simulink library "ammclib_bam_S32K14x"  (R2016a)
settings: Solver=VariableStepAuto  SolverMode=SingleTasking  StartTime=0.0  StopTime=10.0  RelTol=1e-3
undefined symbols (not defined in the file or in its folder): f16A1, f16A2, f16ADCMaxError, f16B0, f16B1, f16B2, f16C1, f16CC1, f16CC1sc, f16CC1sc_D, f16CC1sc_Q, f16CC2, f16CC2sc, f16CC2sc_D, f16CC2sc_Q, f16DerivGain, f16EGain, f16FiltCoef, f16HystOff, f16HystOn, f16IGain, f16IntegGain, f16IntegGainFW, f16IntegGainQ, f16Kd, f16Kq, f16Limit, f16LowerLimit, f16LowerLimit_D, f16LowerLimit_Q, f16LowerLimitFW, f16LowerLimitQ, f16ModIndex, f16OutValOff, f16OutValOn, f16PropGain, f16PropGainFW, f16PropGainQ, f16RampDown, f16RampUp, f16UGain, f16UpperLimit, f16UpperLimit_D, f16UpperLimit_Q, f16UpperLimitFW, f16UpperLimitQ, f16WIGain, f32A1, f32A2, f32ADCMaxError, f32B0, f32B1, f32B2, f32C1, f32CC1, f32CC1sc, f32CC1sc_D, f32CC1sc_Q, f32CC2, f32CC2sc ... (+114)
(part 20 of 22)

== system ammclib_bam_S32K14x/GMCLIB/F16/GMCLIB_DecouplingPMSM_F16 ==
  pUdq : Inport  OutDataTypeStr=Bus: SWLIBS_2Syst_F16  BusOutputAsStruct=on
  pIdq : Inport  Port=2  OutDataTypeStr=Bus: SWLIBS_2Syst_F16  BusOutputAsStruct=on
  f16AngularVel : Inport  Port=3  OutDataTypeStr=int16
  GMCLIB_DecouplingPMSM_SF : S-Function  FunctionName=GMCLIB_DecouplingPMSM_SF_F16  Parameters=showStates,f16Kd,s16KdShift,f16Kq,s16KqShift  SFunctionDeploymentMode=off  EnableBusSupport=off
  copyright : Subsystem
      mask Display: text(10,90,'FILE:');text(10,75,'DESRIPTION:');text(10,60,'COPYRIGHT:');text(10,45,'VERSION:');text(10,30,'DATE:')
  copyright2 : Subsystem
      mask Display: text(10,90,'GMCLIB_DecouplingPMSM_BAM_F16.mdl');text(10,75,'Decoupling of d and q axis of PMSM model.');text(10,60,'NXP 2020');text(10,45,'1.0');text(10,30,'24-Mar-2020');
  f16Kd : Ground
  f16Kq : Ground
  s16KdShift : Ground
  s16KqShift : Ground
  pUdqDec : Outport
  wires:
  GMCLIB_DecouplingPMSM_SF/1 -> pUdqDec/1
  s16KqShift/1 -> GMCLIB_DecouplingPMSM_SF/7
  f16Kq/1 -> GMCLIB_DecouplingPMSM_SF/6
  s16KdShift/1 -> GMCLIB_DecouplingPMSM_SF/5
  f16Kd/1 -> GMCLIB_DecouplingPMSM_SF/4
  f16AngularVel/1 -> GMCLIB_DecouplingPMSM_SF/3
  pIdq/1 -> GMCLIB_DecouplingPMSM_SF/2
  pUdq/1 -> GMCLIB_DecouplingPMSM_SF/1

== system ammclib_bam_S32K14x/GMCLIB/F16/GMCLIB_ElimDcBusRip_F16 ==
  pIn : Inport  OutDataTypeStr=Bus: SWLIBS_2Syst_F16  BusOutputAsStruct=on
  f16ArgDcBusMsr : Inport  Port=2  OutDataTypeStr=int16
  GMCLIB_ElimDcBusRip_SF : S-Function  FunctionName=GMCLIB_ElimDcBusRip_SF_F16  Parameters=showStates,f16ModIndex  SFunctionDeploymentMode=off  EnableBusSupport=off
  copyright : Subsystem
      mask Display: text(10,90,'FILE:');text(10,75,'DESRIPTION:');text(10,60,'COPYRIGHT:');text(10,45,'VERSION:');text(10,30,'DATE:')
  copyright2 : Subsystem
      mask Display: text(10,90,'GMCLIB_ElimDcBusRip_BAM_F16.mdl');text(10,75,'DC Bus voltage ripple elimination function.');text(10,60,'NXP 2020');text(10,45,'1.0');text(10,30,'18-Mar-2020');
  f16ModIndex : Ground
  pOut : Outport
  wires:
  GMCLIB_ElimDcBusRip_SF/1 -> pOut/1
  f16ModIndex/1 -> GMCLIB_ElimDcBusRip_SF/3
  f16ArgDcBusMsr/1 -> GMCLIB_ElimDcBusRip_SF/2
  pIn/1 -> GMCLIB_ElimDcBusRip_SF/1

== system ammclib_bam_S32K14x/GMCLIB/F16/GMCLIB_ParkInv_F16 ==
  pInAngle : Inport  OutDataTypeStr=Bus: SWLIBS_2Syst_F16  BusOutputAsStruct=on
  pIn : Inport  Port=2  OutDataTypeStr=Bus: SWLIBS_2Syst_F16  BusOutputAsStruct=on
  GMCLIB_ParkInv_SF : S-Function  FunctionName=GMCLIB_ParkInv_SF_F16  SFunctionDeploymentMode=off  EnableBusSupport=off
  copyright : Subsystem
      mask Display: text(10,90,'FILE:');text(10,75,'DESRIPTION:');text(10,60,'COPYRIGHT:');text(10,45,'VERSION:');text(10,30,'DATE:')
  copyright2 : Subsystem
      mask Display: text(10,90,'GMCLIB_ParkInv_BAM_F16.mdl');text(10,75,'Inverse Park transformation.');text(10,60,'NXP 2020');text(10,45,'1.0');text(10,30,'18-Mar-2020');
  pOut : Outport
  wires:
  GMCLIB_ParkInv_SF/1 -> pOut/1
  pIn/1 -> GMCLIB_ParkInv_SF/2
  pInAngle/1 -> GMCLIB_ParkInv_SF/1

== system ammclib_bam_S32K14x/GMCLIB/F16/GMCLIB_Park_F16 ==
  pInAngle : Inport  OutDataTypeStr=Bus: SWLIBS_2Syst_F16  BusOutputAsStruct=on
  pIn : Inport  Port=2  OutDataTypeStr=Bus: SWLIBS_2Syst_F16  BusOutputAsStruct=on
  GMCLIB_Park_SF : S-Function  FunctionName=GMCLIB_Park_SF_F16  SFunctionDeploymentMode=off  EnableBusSupport=off
  copyright : Subsystem
      mask Display: text(10,90,'FILE:');text(10,75,'DESRIPTION:');text(10,60,'COPYRIGHT:');text(10,45,'VERSION:');text(10,30,'DATE:')
  copyright2 : Subsystem
      mask Display: text(10,90,'GMCLIB_Park_BAM_F16.mdl');text(10,75,'Park transformation.');text(10,60,'NXP 2020');text(10,45,'1.0');text(10,30,'18-Mar-2020');
  pOut : Outport
  wires:
  GMCLIB_Park_SF/1 -> pOut/1
  pIn/1 -> GMCLIB_Park_SF/2
  pInAngle/1 -> GMCLIB_Park_SF/1

== system ammclib_bam_S32K14x/GMCLIB/F16/GMCLIB_PwmIct_F16 ==
  pIn : Inport  OutDataTypeStr=Bus: SWLIBS_2Syst_F16  BusOutputAsStruct=on
  GMCLIB_PwmIct_SF : S-Function  FunctionName=GMCLIB_PwmIct_SF_F16  SFunctionDeploymentMode=off  EnableBusSupport=off
  copyright : Subsystem
      mask Display: text(10,90,'FILE:');text(10,75,'DESRIPTION:');text(10,60,'COPYRIGHT:');text(10,45,'VERSION:');text(10,30,'DATE:')
  copyright2 : Subsystem
      mask Display: text(10,90,'GMCLIB_PwmIct_BAM_F16.mdl');text(10,75,'General Sinusoidal PWM.');text(10,60,'NXP 2020');text(10,45,'1.0');text(10,30,'18-Mar-2020');
  u16Sector : Outport
  pOut : Outport  Port=2
  wires:
  GMCLIB_PwmIct_SF/2 -> pOut/1
  GMCLIB_PwmIct_SF/1 -> u16Sector/1
  pIn/1 -> GMCLIB_PwmIct_SF/1

== system ammclib_bam_S32K14x/GMCLIB/F16/GMCLIB_SvmSci_F16 ==
  pIn : Inport  OutDataTypeStr=Bus: SWLIBS_2Syst_F16  BusOutputAsStruct=on
  GMCLIB_SvmSci_SF : S-Function  FunctionName=GMCLIB_SvmSci_SF_F16  SFunctionDeploymentMode=off  EnableBusSupport=off
  copyright : Subsystem
      mask Display: text(10,90,'FILE:');text(10,75,'DESRIPTION:');text(10,60,'COPYRIGHT:');text(10,45,'VERSION:');text(10,30,'DATE:')
  copyright2 : Subsystem
      mask Display: text(10,90,'GMCLIB_SvmSci_BAM_F16.mdl');text(10,75,'General Sinusoidal Modulation with Injection of Third Harmonic.');text(10,60,'NXP 2020');text(10,45,'1.0');text(10,30,'18-Mar-2020');
  u16Sector : Outport
  pOut : Outport  Port=2
  wires:
  GMCLIB_SvmSci_SF/2 -> pOut/1
  GMCLIB_SvmSci_SF/1 -> u16Sector/1
  pIn/1 -> GMCLIB_SvmSci_SF/1

== system ammclib_bam_S32K14x/GMCLIB/F16/GMCLIB_SvmStd_F16 ==
  pIn : Inport  OutDataTypeStr=Bus: SWLIBS_2Syst_F16  BusOutputAsStruct=on
  GMCLIB_SvmStd_SF : S-Function  FunctionName=GMCLIB_SvmStd_SF_F16  SFunctionDeploymentMode=off  EnableBusSupport=off
  copyright : Subsystem
      mask Display: text(10,90,'FILE:');text(10,75,'DESRIPTION:');text(10,60,'COPYRIGHT:');text(10,45,'VERSION:');text(10,30,'DATE:')
  copyright2 : Subsystem
      mask Display: text(10,90,'GMCLIB_SvmStd_BAM_F16.mdl');text(10,75,'Standard Space Vector Modulation.');text(10,60,'NXP 2020');text(10,45,'1.0');text(10,30,'18-Mar-2020');
  u16Sector : Outport
  pOut : Outport  Port=2
  wires:
  GMCLIB_SvmStd_SF/2 -> pOut/1
  GMCLIB_SvmStd_SF/1 -> u16Sector/1
  pIn/1 -> GMCLIB_SvmStd_SF/1

== system ammclib_bam_S32K14x/GMCLIB/F16/GMCLIB_SvmU0n_F16 ==
  pIn : Inport  OutDataTypeStr=Bus: SWLIBS_2Syst_F16  BusOutputAsStruct=on
  GMCLIB_SvmU0n_SF : S-Function  FunctionName=GMCLIB_SvmU0n_SF_F16  SFunctionDeploymentMode=off  EnableBusSupport=off
  copyright : Subsystem
      mask Display: text(10,90,'FILE:');text(10,75,'DESRIPTION:');text(10,60,'COPYRIGHT:');text(10,45,'VERSION:');text(10,30,'DATE:')
  copyright2 : Subsystem
      mask Display: text(10,90,'GMCLIB_SvmU0n_BAM_F16.mdl');text(10,75,'Special Space Vector Modulation with O_000 Nulls.');text(10,60,'NXP 2020');text(10,45,'1.0');text(10,30,'18-Mar-2020');
  u16Sector : Outport
  pOut : Outport  Port=2
  wires:
  GMCLIB_SvmU0n_SF/2 -> pOut/1
  GMCLIB_SvmU0n_SF/1 -> u16Sector/1
  pIn/1 -> GMCLIB_SvmU0n_SF/1

== system ammclib_bam_S32K14x/GMCLIB/F16/GMCLIB_SvmU7n_F16 ==
  pIn : Inport  OutDataTypeStr=Bus: SWLIBS_2Syst_F16  BusOutputAsStruct=on
  GMCLIB_SvmU7n_SF : S-Function  FunctionName=GMCLIB_SvmU7n_SF_F16  SFunctionDeploymentMode=off  EnableBusSupport=off
  copyright : Subsystem
      mask Display: text(10,90,'FILE:');text(10,75,'DESRIPTION:');text(10,60,'COPYRIGHT:');text(10,45,'VERSION:');text(10,30,'DATE:')
  copyright2 : Subsystem
      mask Display: text(10,90,'GMCLIB_SvmU7n_BAM_F16.mdl');text(10,75,'Special Space Vector Modulation with O_111 Ones.');text(10,60,'NXP 2020');text(10,45,'1.0');text(10,30,'18-Mar-2020');
  u16Sector : Outport
  pOut : Outport  Port=2
  wires:
  GMCLIB_SvmU7n_SF/2 -> pOut/1
  GMCLIB_SvmU7n_SF/1 -> u16Sector/1
  pIn/1 -> GMCLIB_SvmU7n_SF/1

== system ammclib_bam_S32K14x/GMCLIB/F16/GMCLIB_VRot_F16 ==
  f16InVec : Inport  OutDataTypeStr=Bus: SWLIBS_2Syst_F16  BusOutputAsStruct=on
  f16Angle : Inport  Port=2  OutDataTypeStr=int16
  GMCLIB_VRot_SF : S-Function  FunctionName=GMCLIB_VRot_SF_F16  SFunctionDeploymentMode=off  EnableBusSupport=off
  copyright : Subsystem
      mask Display: text(10,90,'FILE:');text(10,75,'DESRIPTION:');text(10,60,'COPYRIGHT:');text(10,45,'VERSION:');text(10,30,'DATE:')
  copyright2 : Subsystem
      mask Display: text(10,90,'GMCLIB_VRot_BAM_F16.mdl');text(10,75,'Vector rotation.');text(10,60,'NXP 2020');text(10,45,'1.0');text(10,30,'05-Jun-2020');
  f16OutVec : Outport
  wires:
  GMCLIB_VRot_SF/1 -> f16OutVec/1
  f16Angle/1 -> GMCLIB_VRot_SF/2
  f16InVec/1 -> GMCLIB_VRot_SF/1

== system ammclib_bam_S32K14x/GMCLIB/F16/GMCLIB_VUnit_F16 ==
  f16InVec : Inport  OutDataTypeStr=Bus: SWLIBS_2Syst_F16  BusOutputAsStruct=on
  GMCLIB_VUnit_SF : S-Function  FunctionName=GMCLIB_VUnit_SF_F16  SFunctionDeploymentMode=off  EnableBusSupport=off
  copyright : Subsystem
      mask Display: text(10,90,'FILE:');text(10,75,'DESRIPTION:');text(10,60,'COPYRIGHT:');text(10,45,'VERSION:');text(10,30,'DATE:')
  copyright2 : Subsystem
      mask Display: text(10,90,'GMCLIB_VUnit_BAM_F16.mdl');text(10,75,'Vector normalization.');text(10,60,'NXP 2020');text(10,45,'1.0');text(10,30,'08-Jun-2020');
  f16OutVec : Outport
  wires:
  GMCLIB_VUnit_SF/1 -> f16OutVec/1
  f16InVec/1 -> GMCLIB_VUnit_SF/1

== system ammclib_bam_S32K14x/GMCLIB/F16/GMCLIB_Vpol2xy_F16 ==
  f16InVec : Inport  OutDataTypeStr=Bus: SWLIBS_2Syst_F16  BusOutputAsStruct=on
  GMCLIB_Vpol2xy_SF : S-Function  FunctionName=GMCLIB_Vpol2xy_SF_F16  SFunctionDeploymentMode=off  EnableBusSupport=off
  copyright : Subsystem
      mask Display: text(10,90,'FILE:');text(10,75,'DESRIPTION:');text(10,60,'COPYRIGHT:');text(10,45,'VERSION:');text(10,30,'DATE:')
  copyright2 : Subsystem
      mask Display: text(10,90,'GMCLIB_Vpol2xy_BAM_F16.mdl');text(10,75,'Transformation of polar coordinate system to Cartesian.');text(10,60,'NXP 2020');text(10,45,'1.0');text(10,30,'10-Jun-2020');
  f16OutVec : Outport
  wires:
  GMCLIB_Vpol2xy_SF/1 -> f16OutVec/1
  f16InVec/1 -> GMCLIB_Vpol2xy_SF/1

== system ammclib_bam_S32K14x/GMCLIB/F16/GMCLIB_Vxy2pol_F16 ==
  f16InVec : Inport  OutDataTypeStr=Bus: SWLIBS_2Syst_F16  BusOutputAsStruct=on
  GMCLIB_Vxy2pol_SF : S-Function  FunctionName=GMCLIB_Vxy2pol_SF_F16  SFunctionDeploymentMode=off  EnableBusSupport=off
  copyright : Subsystem
      mask Display: text(10,90,'FILE:');text(10,75,'DESRIPTION:');text(10,60,'COPYRIGHT:');text(10,45,'VERSION:');text(10,30,'DATE:')
  copyright2 : Subsystem
      mask Display: text(10,90,'GMCLIB_Vxy2pol_BAM_F16.mdl');text(10,75,'Transformation of Cartesian coordinate system to polar.');text(10,60,'NXP 2020');text(10,45,'1.0');text(10,30,'11-Jun-2020');
  f16OutVec : Outport
  wires:
  GMCLIB_Vxy2pol_SF/1 -> f16OutVec/1
  f16InVec/1 -> GMCLIB_Vxy2pol_SF/1

== system ammclib_bam_S32K14x/GMCLIB/F32/GMCLIB_BetaProjection3Ph_F32 ==
  pIn : Inport  OutDataTypeStr=Bus: SWLIBS_3Syst_F32  BusOutputAsStruct=on
  GMCLIB_BetaProjection3Ph_SF : S-Function  FunctionName=GMCLIB_BetaProjection3Ph_SF_F32  SFunctionDeploymentMode=off  EnableBusSupport=off
  copyright : Subsystem
      mask Display: text(10,90,'FILE:');text(10,75,'DESRIPTION:');text(10,60,'COPYRIGHT:');text(10,45,'VERSION:');text(10,30,'DATE:')
  copyright2 : Subsystem
      mask Display: text(10,90,'GMCLIB_BetaProjection3Ph_BAM_F32.mdl');text(10,75,'3-phase Beta-projection transformation.');text(10,60,'NXP 2020');text(10,45,'1.0');text(10,30,'18-Mar-2020');
  pOut : Outport
  wires:
  GMCLIB_BetaProjection3Ph_SF/1 -> pOut/1
  pIn/1 -> GMCLIB_BetaProjection3Ph_SF/1

== system ammclib_bam_S32K14x/GMCLIB/F32/GMCLIB_BetaProjection_F32 ==
  pIn : Inport  OutDataTypeStr=Bus: SWLIBS_3Syst_F32  BusOutputAsStruct=on
  GMCLIB_BetaProjection_SF : S-Function  FunctionName=GMCLIB_BetaProjection_SF_F32  SFunctionDeploymentMode=off  EnableBusSupport=off
  copyright : Subsystem
      mask Display: text(10,90,'FILE:');text(10,75,'DESRIPTION:');text(10,60,'COPYRIGHT:');text(10,45,'VERSION:');text(10,30,'DATE:')
  copyright2 : Subsystem
      mask Display: text(10,90,'GMCLIB_BetaProjection_BAM_F32.mdl');text(10,75,'Beta Projection transformation.');text(10,60,'NXP 2020');text(10,45,'1.0');text(10,30,'18-Mar-2020');
  pOut : Outport
  wires:
  GMCLIB_BetaProjection_SF/1 -> pOut/1
  pIn/1 -> GMCLIB_BetaProjection_SF/1

== system ammclib_bam_S32K14x/GMCLIB/F32/GMCLIB_ClarkInv_F32 ==
  pIn : Inport  OutDataTypeStr=Bus: SWLIBS_2Syst_F32  BusOutputAsStruct=on
  GMCLIB_ClarkInv_SF : S-Function  FunctionName=GMCLIB_ClarkInv_SF_F32  SFunctionDeploymentMode=off  EnableBusSupport=off
  copyright : Subsystem
      mask Display: text(10,90,'FILE:');text(10,75,'DESRIPTION:');text(10,60,'COPYRIGHT:');text(10,45,'VERSION:');text(10,30,'DATE:')
  copyright2 : Subsystem
      mask Display: text(10,90,'GMCLIB_ClarkInv_BAM_F32.mdl');text(10,75,'Inverse Clarke transformation');text(10,60,'NXP 2020');text(10,45,'1.0');text(10,30,'18-Mar-2020');
  pOut : Outport
  wires:
  GMCLIB_ClarkInv_SF/1 -> pOut/1
  pIn/1 -> GMCLIB_ClarkInv_SF/1

== system ammclib_bam_S32K14x/GMCLIB/F32/GMCLIB_Clark_F32 ==
  pIn : Inport  OutDataTypeStr=Bus: SWLIBS_3Syst_F32  BusOutputAsStruct=on
  GMCLIB_Clark_SF : S-Function  FunctionName=GMCLIB_Clark_SF_F32  SFunctionDeploymentMode=off  EnableBusSupport=off
  copyright : Subsystem
      mask Display: text(10,90,'FILE:');text(10,75,'DESRIPTION:');text(10,60,'COPYRIGHT:');text(10,45,'VERSION:');text(10,30,'DATE:')
  copyright2 : Subsystem
      mask Display: text(10,90,'GMCLIB_Clark_BAM_F32.mdl');text(10,75,'Clarke transformation.');text(10,60,'NXP 2020');text(10,45,'1.0');text(10,30,'18-Mar-2020');
  pOut : Outport
  wires:
  GMCLIB_Clark_SF/1 -> pOut/1
  pIn/1 -> GMCLIB_Clark_SF/1

== system ammclib_bam_S32K14x/GMCLIB/F32/GMCLIB_DecouplingPMSM_F32 ==
  pUdq : Inport  OutDataTypeStr=Bus: SWLIBS_2Syst_F32  BusOutputAsStruct=on
  pIdq : Inport  Port=2  OutDataTypeStr=Bus: SWLIBS_2Syst_F32  BusOutputAsStruct=on
  f32AngularVel : Inport  Port=3  OutDataTypeStr=int32
  GMCLIB_DecouplingPMSM_SF : S-Function  FunctionName=GMCLIB_DecouplingPMSM_SF_F32  Parameters=showStates,f32Kd,s16KdShift,f32Kq,s16KqShift  SFunctionDeploymentMode=off  EnableBusSupport=off
  copyright : Subsystem
      mask Display: text(10,90,'FILE:');text(10,75,'DESRIPTION:');text(10,60,'COPYRIGHT:');text(10,45,'VERSION:');text(10,30,'DATE:')
  copyright2 : Subsystem
      mask Display: text(10,90,'GMCLIB_DecouplingPMSM_BAM_F32.mdl');text(10,75,'Decoupling of d and q axis of PMSM model.');text(10,60,'NXP 2020');text(10,45,'1.0');text(10,30,'24-Mar-2020');
  f32Kd : Ground
  f32Kq : Ground
  s16KdShift : Ground
  s16KqShift : Ground
  pUdqDec : Outport
  wires:
  GMCLIB_DecouplingPMSM_SF/1 -> pUdqDec/1
  s16KqShift/1 -> GMCLIB_DecouplingPMSM_SF/7
  f32Kq/1 -> GMCLIB_DecouplingPMSM_SF/6
  s16KdShift/1 -> GMCLIB_DecouplingPMSM_SF/5
  f32Kd/1 -> GMCLIB_DecouplingPMSM_SF/4
  f32AngularVel/1 -> GMCLIB_DecouplingPMSM_SF/3
  pIdq/1 -> GMCLIB_DecouplingPMSM_SF/2
  pUdq/1 -> GMCLIB_DecouplingPMSM_SF/1

== system ammclib_bam_S32K14x/GMCLIB/F32/GMCLIB_ElimDcBusRip_F32 ==
  pIn : Inport  OutDataTypeStr=Bus: SWLIBS_2Syst_F32  BusOutputAsStruct=on
  f32ArgDcBusMsr : Inport  Port=2  OutDataTypeStr=int32
  GMCLIB_ElimDcBusRip_SF : S-Function  FunctionName=GMCLIB_ElimDcBusRip_SF_F32  Parameters=showStates,f32ModIndex  SFunctionDeploymentMode=off  EnableBusSupport=off
  copyright : Subsystem
      mask Display: text(10,90,'FILE:');text(10,75,'DESRIPTION:');text(10,60,'COPYRIGHT:');text(10,45,'VERSION:');text(10,30,'DATE:')
  copyright2 : Subsystem
      mask Display: text(10,90,'GMCLIB_ElimDcBusRip_BAM_F32.mdl');text(10,75,'DC Bus voltage ripple elimination function.');text(10,60,'NXP 2020');text(10,45,'1.0');text(10,30,'18-Mar-2020');
  f32ModIndex : Ground
  pOut : Outport
  wires:
  GMCLIB_ElimDcBusRip_SF/1 -> pOut/1
  f32ModIndex/1 -> GMCLIB_ElimDcBusRip_SF/3
  f32ArgDcBusMsr/1 -> GMCLIB_ElimDcBusRip_SF/2
  pIn/1 -> GMCLIB_ElimDcBusRip_SF/1

== system ammclib_bam_S32K14x/GMCLIB/F32/GMCLIB_ParkInv_F32 ==
  pInAngle : Inport  OutDataTypeStr=Bus: SWLIBS_2Syst_F32  BusOutputAsStruct=on
  pIn : Inport  Port=2  OutDataTypeStr=Bus: SWLIBS_2Syst_F32  BusOutputAsStruct=on
  GMCLIB_ParkInv_SF : S-Function  FunctionName=GMCLIB_ParkInv_SF_F32  SFunctionDeploymentMode=off  EnableBusSupport=off
  copyright : Subsystem
      mask Display: text(10,90,'FILE:');text(10,75,'DESRIPTION:');text(10,60,'COPYRIGHT:');text(10,45,'VERSION:');text(10,30,'DATE:')
  copyright2 : Subsystem
      mask Display: text(10,90,'GMCLIB_ParkInv_BAM_F32.mdl');text(10,75,'Inverse Park transformation.');text(10,60,'NXP 2020');text(10,45,'1.0');text(10,30,'18-Mar-2020');
  pOut : Outport
  wires:
  GMCLIB_ParkInv_SF/1 -> pOut/1
  pIn/1 -> GMCLIB_ParkInv_SF/2
  pInAngle/1 -> GMCLIB_ParkInv_SF/1

== system ammclib_bam_S32K14x/GMCLIB/F32/GMCLIB_Park_F32 ==
  pInAngle : Inport  OutDataTypeStr=Bus: SWLIBS_2Syst_F32  BusOutputAsStruct=on
  pIn : Inport  Port=2  OutDataTypeStr=Bus: SWLIBS_2Syst_F32  BusOutputAsStruct=on
  GMCLIB_Park_SF : S-Function  FunctionName=GMCLIB_Park_SF_F32  SFunctionDeploymentMode=off  EnableBusSupport=off
  copyright : Subsystem
      mask Display: text(10,90,'FILE:');text(10,75,'DESRIPTION:');text(10,60,'COPYRIGHT:');text(10,45,'VERSION:');text(10,30,'DATE:')
  copyright2 : Subsystem
      mask Display: text(10,90,'GMCLIB_Park_BAM_F32.mdl');text(10,75,'Park transformation.');text(10,60,'NXP 2020');text(10,45,'1.0');text(10,30,'18-Mar-2020');
  pOut : Outport
  wires:
  GMCLIB_Park_SF/1 -> pOut/1
  pIn/1 -> GMCLIB_Park_SF/2
  pInAngle/1 -> GMCLIB_Park_SF/1

== system ammclib_bam_S32K14x/GMCLIB/F32/GMCLIB_PwmIct_F32 ==
  pIn : Inport  OutDataTypeStr=Bus: SWLIBS_2Syst_F32  BusOutputAsStruct=on
  GMCLIB_PwmIct_SF : S-Function  FunctionName=GMCLIB_PwmIct_SF_F32  SFunctionDeploymentMode=off  EnableBusSupport=off
  copyright : Subsystem
      mask Display: text(10,90,'FILE:');text(10,75,'DESRIPTION:');text(10,60,'COPYRIGHT:');text(10,45,'VERSION:');text(10,30,'DATE:')
  copyright2 : Subsystem
      mask Display: text(10,90,'GMCLIB_PwmIct_BAM_F32.mdl');text(10,75,'General Sinusoidal PWM.');text(10,60,'NXP 2020');text(10,45,'1.0');text(10,30,'18-Mar-2020');
  u32Sector : Outport
  pOut : Outport  Port=2
  wires:
  GMCLIB_PwmIct_SF/2 -> pOut/1
  GMCLIB_PwmIct_SF/1 -> u32Sector/1
  pIn/1 -> GMCLIB_PwmIct_SF/1

== system ammclib_bam_S32K14x/GMCLIB/F32/GMCLIB_SvmSci_F32 ==
  pIn : Inport  OutDataTypeStr=Bus: SWLIBS_2Syst_F32  BusOutputAsStruct=on
  GMCLIB_SvmSci_SF : S-Function  FunctionName=GMCLIB_SvmSci_SF_F32  SFunctionDeploymentMode=off  EnableBusSupport=off
  copyright : Subsystem
      mask Display: text(10,90,'FILE:');text(10,75,'DESRIPTION:');text(10,60,'COPYRIGHT:');text(10,45,'VERSION:');text(10,30,'DATE:')
  copyright2 : Subsystem
      mask Display: text(10,90,'GMCLIB_SvmSci_BAM_F32.mdl');text(10,75,'General Sinusoidal Modulation with Injection of Third Harmonic.');text(10,60,'NXP 2020');text(10,45,'1.0');text(10,30,'18-Mar-2020');
  u32Sector : Outport
  pOut : Outport  Port=2
  wires:
  GMCLIB_SvmSci_SF/2 -> pOut/1
  GMCLIB_SvmSci_SF/1 -> u32Sector/1
  pIn/1 -> GMCLIB_SvmSci_SF/1

== system ammclib_bam_S32K14x/GMCLIB/F32/GMCLIB_SvmStd_F32 ==
  pIn : Inport  OutDataTypeStr=Bus: SWLIBS_2Syst_F32  BusOutputAsStruct=on
  GMCLIB_SvmStd_SF : S-Function  FunctionName=GMCLIB_SvmStd_SF_F32  SFunctionDeploymentMode=off  EnableBusSupport=off
  copyright : Subsystem
      mask Display: text(10,90,'FILE:');text(10,75,'DESRIPTION:');text(10,60,'COPYRIGHT:');text(10,45,'VERSION:');text(10,30,'DATE:')
  copyright2 : Subsystem
      mask Display: text(10,90,'GMCLIB_SvmStd_BAM_F32.mdl');text(10,75,'Standard Space Vector Modulation.');text(10,60,'NXP 2020');text(10,45,'1.0');text(10,30,'18-Mar-2020');
  u32Sector : Outport
  pOut : Outport  Port=2
  wires:
  GMCLIB_SvmStd_SF/2 -> pOut/1
  GMCLIB_SvmStd_SF/1 -> u32Sector/1
  pIn/1 -> GMCLIB_SvmStd_SF/1

== system ammclib_bam_S32K14x/GMCLIB/F32/GMCLIB_SvmU0n_F32 ==
  pIn : Inport  OutDataTypeStr=Bus: SWLIBS_2Syst_F32  BusOutputAsStruct=on
  GMCLIB_SvmU0n_SF : S-Function  FunctionName=GMCLIB_SvmU0n_SF_F32  SFunctionDeploymentMode=off  EnableBusSupport=off
  copyright : Subsystem
      mask Display: text(10,90,'FILE:');text(10,75,'DESRIPTION:');text(10,60,'COPYRIGHT:');text(10,45,'VERSION:');text(10,30,'DATE:')
  copyright2 : Subsystem
      mask Display: text(10,90,'GMCLIB_SvmU0n_BAM_F32.mdl');text(10,75,'Special Space Vector Modulation with O_000 Nulls.');text(10,60,'NXP 2020');text(10,45,'1.0');text(10,30,'18-Mar-2020');
  u32Sector : Outport
  pOut : Outport  Port=2
  wires:
  GMCLIB_SvmU0n_SF/2 -> pOut/1
  GMCLIB_SvmU0n_SF/1 -> u32Sector/1
  pIn/1 -> GMCLIB_SvmU0n_SF/1

== system ammclib_bam_S32K14x/GMCLIB/F32/GMCLIB_SvmU7n_F32 ==
  pIn : Inport  OutDataTypeStr=Bus: SWLIBS_2Syst_F32  BusOutputAsStruct=on
  GMCLIB_SvmU7n_SF : S-Function  FunctionName=GMCLIB_SvmU7n_SF_F32  SFunctionDeploymentMode=off  EnableBusSupport=off
  copyright : Subsystem
      mask Display: text(10,90,'FILE:');text(10,75,'DESRIPTION:');text(10,60,'COPYRIGHT:');text(10,45,'VERSION:');text(10,30,'DATE:')
  copyright2 : Subsystem
      mask Display: text(10,90,'GMCLIB_SvmU7n_BAM_F32.mdl');text(10,75,'Special Space Vector Modulation with O_111 Ones.');text(10,60,'NXP 2020');text(10,45,'1.0');text(10,30,'18-Mar-2020');
  u32Sector : Outport
  pOut : Outport  Port=2
  wires:
  GMCLIB_SvmU7n_SF/2 -> pOut/1
  GMCLIB_SvmU7n_SF/1 -> u32Sector/1
  pIn/1 -> GMCLIB_SvmU7n_SF/1

== system ammclib_bam_S32K14x/GMCLIB/F32/GMCLIB_VRot_F32 ==
  f32InVec : Inport  OutDataTypeStr=Bus: SWLIBS_2Syst_F32  BusOutputAsStruct=on
  f32Angle : Inport  Port=2  OutDataTypeStr=int32
  GMCLIB_VRot_SF : S-Function  FunctionName=GMCLIB_VRot_SF_F32  SFunctionDeploymentMode=off  EnableBusSupport=off
  copyright : Subsystem
      mask Display: text(10,90,'FILE:');text(10,75,'DESRIPTION:');text(10,60,'COPYRIGHT:');text(10,45,'VERSION:');text(10,30,'DATE:')
  copyright2 : Subsystem
      mask Display: text(10,90,'GMCLIB_VRot_BAM_F32.mdl');text(10,75,'Vector rotation.');text(10,60,'NXP 2020');text(10,45,'1.0');text(10,30,'05-Jun-2020');
  f32OutVec : Outport
  wires:
  GMCLIB_VRot_SF/1 -> f32OutVec/1
  f32Angle/1 -> GMCLIB_VRot_SF/2
  f32InVec/1 -> GMCLIB_VRot_SF/1

== system ammclib_bam_S32K14x/GMCLIB/F32/GMCLIB_VUnit_F32 ==
  f32InVec : Inport  OutDataTypeStr=Bus: SWLIBS_2Syst_F32  BusOutputAsStruct=on
  GMCLIB_VUnit_SF : S-Function  FunctionName=GMCLIB_VUnit_SF_F32  SFunctionDeploymentMode=off  EnableBusSupport=off
  copyright : Subsystem
      mask Display: text(10,90,'FILE:');text(10,75,'DESRIPTION:');text(10,60,'COPYRIGHT:');text(10,45,'VERSION:');text(10,30,'DATE:')
  copyright2 : Subsystem
      mask Display: text(10,90,'GMCLIB_VUnit_BAM_F32.mdl');text(10,75,'Vector normalization.');text(10,60,'NXP 2020');text(10,45,'1.0');text(10,30,'08-Jun-2020');
  f32OutVec : Outport
  wires:
  GMCLIB_VUnit_SF/1 -> f32OutVec/1
  f32InVec/1 -> GMCLIB_VUnit_SF/1

== system ammclib_bam_S32K14x/GMCLIB/F32/GMCLIB_Vpol2xy_F32 ==
  f32InVec : Inport  OutDataTypeStr=Bus: SWLIBS_2Syst_F32  BusOutputAsStruct=on
  GMCLIB_Vpol2xy_SF : S-Function  FunctionName=GMCLIB_Vpol2xy_SF_F32  SFunctionDeploymentMode=off  EnableBusSupport=off
  copyright : Subsystem
      mask Display: text(10,90,'FILE:');text(10,75,'DESRIPTION:');text(10,60,'COPYRIGHT:');text(10,45,'VERSION:');text(10,30,'DATE:')
  copyright2 : Subsystem
      mask Display: text(10,90,'GMCLIB_Vpol2xy_BAM_F32.mdl');text(10,75,'Transformation of polar coordinate system to Cartesian.');text(10,60,'NXP 2020');text(10,45,'1.0');text(10,30,'10-Jun-2020');
  f32OutVec : Outport
  wires:
  GMCLIB_Vpol2xy_SF/1 -> f32OutVec/1
  f32InVec/1 -> GMCLIB_Vpol2xy_SF/1

== system ammclib_bam_S32K14x/GMCLIB/F32/GMCLIB_Vxy2pol_F32 ==
  f32InVec : Inport  OutDataTypeStr=Bus: SWLIBS_2Syst_F32  BusOutputAsStruct=on
  GMCLIB_Vxy2pol_SF : S-Function  FunctionName=GMCLIB_Vxy2pol_SF_F32  SFunctionDeploymentMode=off  EnableBusSupport=off
  copyright : Subsystem
      mask Display: text(10,90,'FILE:');text(10,75,'DESRIPTION:');text(10,60,'COPYRIGHT:');text(10,45,'VERSION:');text(10,30,'DATE:')
  copyright2 : Subsystem
      mask Display: text(10,90,'GMCLIB_Vxy2pol_BAM_F32.mdl');text(10,75,'Transformation of Cartesian coordinate system to polar.');text(10,60,'NXP 2020');text(10,45,'1.0');text(10,30,'11-Jun-2020');
  f32OutVec : Outport
  wires:
  GMCLIB_Vxy2pol_SF/1 -> f32OutVec/1
  f32InVec/1 -> GMCLIB_Vxy2pol_SF/1

== system ammclib_bam_S32K14x/GMCLIB/FLT/GMCLIB_BetaProjection3Ph_FLT ==
  pIn : Inport  OutDataTypeStr=Bus: SWLIBS_3Syst_FLT  BusOutputAsStruct=on
  GMCLIB_BetaProjection3Ph_SF : S-Function  FunctionName=GMCLIB_BetaProjection3Ph_SF_FLT  SFunctionDeploymentMode=off  EnableBusSupport=off
  copyright : Subsystem
      mask Display: text(10,90,'FILE:');text(10,75,'DESRIPTION:');text(10,60,'COPYRIGHT:');text(10,45,'VERSION:');text(10,30,'DATE:')
  copyright2 : Subsystem
      mask Display: text(10,90,'GMCLIB_BetaProjection3Ph_BAM_FLT.mdl');text(10,75,'Beta Projection transformation.');text(10,60,'NXP 2020');text(10,45,'1.0');text(10,30,'18-Mar-2020');
  pOut : Outport
  wires:
  GMCLIB_BetaProjection3Ph_SF/1 -> pOut/1
  pIn/1 -> GMCLIB_BetaProjection3Ph_SF/1

== system ammclib_bam_S32K14x/GMCLIB/FLT/GMCLIB_BetaProjection_FLT ==
  pIn : Inport  OutDataTypeStr=Bus: SWLIBS_3Syst_FLT  BusOutputAsStruct=on
  GMCLIB_BetaProjection_SF : S-Function  FunctionName=GMCLIB_BetaProjection_SF_FLT  SFunctionDeploymentMode=off  EnableBusSupport=off
  copyright : Subsystem
      mask Display: text(10,90,'FILE:');text(10,75,'DESRIPTION:');text(10,60,'COPYRIGHT:');text(10,45,'VERSION:');text(10,30,'DATE:')
  copyright2 : Subsystem
      mask Display: text(10,90,'GMCLIB_BetaProjection_BAM_FLT.mdl');text(10,75,'Beta Projection transformation.');text(10,60,'NXP 2020');text(10,45,'1.0');text(10,30,'18-Mar-2020');
  pOut : Outport
  wires:
  GMCLIB_BetaProjection_SF/1 -> pOut/1
  pIn/1 -> GMCLIB_BetaProjection_SF/1

== system ammclib_bam_S32K14x/GMCLIB/FLT/GMCLIB_ClarkInv_FLT ==
  pIn : Inport  OutDataTypeStr=Bus: SWLIBS_2Syst_FLT  BusOutputAsStruct=on
  GMCLIB_ClarkInv_SF : S-Function  FunctionName=GMCLIB_ClarkInv_SF_FLT  SFunctionDeploymentMode=off  EnableBusSupport=off
  copyright : Subsystem
      mask Display: text(10,90,'FILE:');text(10,75,'DESRIPTION:');text(10,60,'COPYRIGHT:');text(10,45,'VERSION:');text(10,30,'DATE:')
  copyright2 : Subsystem
      mask Display: text(10,90,'GMCLIB_ClarkInv_BAM_FLT.mdl');text(10,75,'Inverse Clarke transformation');text(10,60,'NXP 2020');text(10,45,'1.0');text(10,30,'18-Mar-2020');
  pOut : Outport
  wires:
  GMCLIB_ClarkInv_SF/1 -> pOut/1
  pIn/1 -> GMCLIB_ClarkInv_SF/1

== system ammclib_bam_S32K14x/GMCLIB/FLT/GMCLIB_Clark_FLT ==
  pIn : Inport  OutDataTypeStr=Bus: SWLIBS_3Syst_FLT  BusOutputAsStruct=on
  GMCLIB_Clark_SF : S-Function  FunctionName=GMCLIB_Clark_SF_FLT  SFunctionDeploymentMode=off  EnableBusSupport=off
  copyright : Subsystem
      mask Display: text(10,90,'FILE:');text(10,75,'DESRIPTION:');text(10,60,'COPYRIGHT:');text(10,45,'VERSION:');text(10,30,'DATE:')
  copyright2 : Subsystem
      mask Display: text(10,90,'GMCLIB_Clark_BAM_FLT.mdl');text(10,75,'Clarke transformation.');text(10,60,'NXP 2020');text(10,45,'1.0');text(10,30,'18-Mar-2020');
  pOut : Outport
  wires:
  GMCLIB_Clark_SF/1 -> pOut/1
  pIn/1 -> GMCLIB_Clark_SF/1

== system ammclib_bam_S32K14x/GMCLIB/FLT/GMCLIB_DecouplingPMSM_FLT ==
  pUdq : Inport  OutDataTypeStr=Bus: SWLIBS_2Syst_FLT  BusOutputAsStruct=on
  pIdq : Inport  Port=2  OutDataTypeStr=Bus: SWLIBS_2Syst_FLT  BusOutputAsStruct=on
  fltAngularVel : Inport  Port=3  OutDataTypeStr=single
  GMCLIB_DecouplingPMSM_SF : S-Function  FunctionName=GMCLIB_DecouplingPMSM_SF_FLT  Parameters=showStates,fltLD,fltLQ  SFunctionDeploymentMode=off  EnableBusSupport=off
  copyright : Subsystem
      mask Display: text(10,90,'FILE:');text(10,75,'DESRIPTION:');text(10,60,'COPYRIGHT:');text(10,45,'VERSION:');text(10,30,'DATE:')
  copyright2 : Subsystem
      mask Display: text(10,90,'GMCLIB_DecouplingPMSM_BAM_FLT.mdl');text(10,75,'Decoupling of d and q axis of PMSM model.');text(10,60,'NXP 2020');text(10,45,'1.0');text(10,30,'24-Mar-2020');
  fltLD : Ground
  fltLQ : Ground
  pUdqDec : Outport
  wires:
  GMCLIB_DecouplingPMSM_SF/1 -> pUdqDec/1
  fltLQ/1 -> GMCLIB_DecouplingPMSM_SF/5
  fltLD/1 -> GMCLIB_DecouplingPMSM_SF/4
  fltAngularVel/1 -> GMCLIB_DecouplingPMSM_SF/3
  pIdq/1 -> GMCLIB_DecouplingPMSM_SF/2
  pUdq/1 -> GMCLIB_DecouplingPMSM_SF/1

== system ammclib_bam_S32K14x/GMCLIB/FLT/GMCLIB_ElimDcBusRip_FLT ==
  pIn : Inport  OutDataTypeStr=Bus: SWLIBS_2Syst_FLT  BusOutputAsStruct=on
  fltArgDcBusMsr : Inport  Port=2  OutDataTypeStr=single
  GMCLIB_ElimDcBusRip_SF : S-Function  FunctionName=GMCLIB_ElimDcBusRip_SF_FLT  Parameters=showStates,fltModIndex  SFunctionDeploymentMode=off  EnableBusSupport=off
  copyright : Subsystem
      mask Display: text(10,90,'FILE:');text(10,75,'DESRIPTION:');text(10,60,'COPYRIGHT:');text(10,45,'VERSION:');text(10,30,'DATE:')
  copyright2 : Subsystem
      mask Display: text(10,90,'GMCLIB_ElimDcBusRip_BAM_FLT.mdl');text(10,75,'DC Bus voltage ripple elimination function.');text(10,60,'NXP 2020');text(10,45,'1.0');text(10,30,'18-Mar-2020');
  fltModIndex : Ground
  pOut : Outport
  wires:
  GMCLIB_ElimDcBusRip_SF/1 -> pOut/1
  fltModIndex/1 -> GMCLIB_ElimDcBusRip_SF/3
  fltArgDcBusMsr/1 -> GMCLIB_ElimDcBusRip_SF/2
  pIn/1 -> GMCLIB_ElimDcBusRip_SF/1

== system ammclib_bam_S32K14x/GMCLIB/FLT/GMCLIB_ParkInv_FLT ==
  pInAngle : Inport  OutDataTypeStr=Bus: SWLIBS_2Syst_FLT  BusOutputAsStruct=on
  pIn : Inport  Port=2  OutDataTypeStr=Bus: SWLIBS_2Syst_FLT  BusOutputAsStruct=on
  GMCLIB_ParkInv_SF : S-Function  FunctionName=GMCLIB_ParkInv_SF_FLT  SFunctionDeploymentMode=off  EnableBusSupport=off
  copyright : Subsystem
      mask Display: text(10,90,'FILE:');text(10,75,'DESRIPTION:');text(10,60,'COPYRIGHT:');text(10,45,'VERSION:');text(10,30,'DATE:')
  copyright2 : Subsystem
      mask Display: text(10,90,'GMCLIB_ParkInv_BAM_FLT.mdl');text(10,75,'Inverse Park transformation.');text(10,60,'NXP 2020');text(10,45,'1.0');text(10,30,'18-Mar-2020');
  pOut : Outport
  wires:
  GMCLIB_ParkInv_SF/1 -> pOut/1
  pIn/1 -> GMCLIB_ParkInv_SF/2
  pInAngle/1 -> GMCLIB_ParkInv_SF/1

== system ammclib_bam_S32K14x/GMCLIB/FLT/GMCLIB_Park_FLT ==
  pInAngle : Inport  OutDataTypeStr=Bus: SWLIBS_2Syst_FLT  BusOutputAsStruct=on
  pIn : Inport  Port=2  OutDataTypeStr=Bus: SWLIBS_2Syst_FLT  BusOutputAsStruct=on
  GMCLIB_Park_SF : S-Function  FunctionName=GMCLIB_Park_SF_FLT  SFunctionDeploymentMode=off  EnableBusSupport=off
  copyright : Subsystem
      mask Display: text(10,90,'FILE:');text(10,75,'DESRIPTION:');text(10,60,'COPYRIGHT:');text(10,45,'VERSION:');text(10,30,'DATE:')
  copyright2 : Subsystem
      mask Display: text(10,90,'GMCLIB_Park_BAM_FLT.mdl');text(10,75,'Park transformation.');text(10,60,'NXP 2020');text(10,45,'1.0');text(10,30,'18-Mar-2020');
  pOut : Outport
  wires:
  GMCLIB_Park_SF/1 -> pOut/1
  pIn/1 -> GMCLIB_Park_SF/2
  pInAngle/1 -> GMCLIB_Park_SF/1

== system ammclib_bam_S32K14x/GMCLIB/FLT/GMCLIB_PwmIct_FLT ==
  pIn : Inport  OutDataTypeStr=Bus: SWLIBS_2Syst_FLT  BusOutputAsStruct=on
  GMCLIB_PwmIct_SF : S-Function  FunctionName=GMCLIB_PwmIct_SF_FLT  SFunctionDeploymentMode=off  EnableBusSupport=off
  copyright : Subsystem
      mask Display: text(10,90,'FILE:');text(10,75,'DESRIPTION:');text(10,60,'COPYRIGHT:');text(10,45,'VERSION:');text(10,30,'DATE:')
  copyright2 : Subsystem
      mask Display: text(10,90,'GMCLIB_PwmIct_BAM_FLT.mdl');text(10,75,'General Sinusoidal PWM.');text(10,60,'NXP 2020');text(10,45,'1.0');text(10,30,'18-Mar-2020');
  u32Sector : Outport
  pOut : Outport  Port=2
  wires:
  GMCLIB_PwmIct_SF/2 -> pOut/1
  GMCLIB_PwmIct_SF/1 -> u32Sector/1
  pIn/1 -> GMCLIB_PwmIct_SF/1

== system ammclib_bam_S32K14x/GMCLIB/FLT/GMCLIB_SvmSci_FLT ==
  pIn : Inport  OutDataTypeStr=Bus: SWLIBS_2Syst_FLT  BusOutputAsStruct=on
  GMCLIB_SvmSci_SF : S-Function  FunctionName=GMCLIB_SvmSci_SF_FLT  SFunctionDeploymentMode=off  EnableBusSupport=off
  copyright : Subsystem
      mask Display: text(10,90,'FILE:');text(10,75,'DESRIPTION:');text(10,60,'COPYRIGHT:');text(10,45,'VERSION:');text(10,30,'DATE:')
  copyright2 : Subsystem
      mask Display: text(10,90,'GMCLIB_SvmSci_BAM_FLT.mdl');text(10,75,'General Sinusoidal Modulation with Injection of Third Harmonic.');text(10,60,'NXP 2020');text(10,45,'1.0');text(10,30,'18-Mar-2020');
  u32Sector : Outport
  pOut : Outport  Port=2
  wires:
  GMCLIB_SvmSci_SF/2 -> pOut/1
  GMCLIB_SvmSci_SF/1 -> u32Sector/1
  pIn/1 -> GMCLIB_SvmSci_SF/1

== system ammclib_bam_S32K14x/GMCLIB/FLT/GMCLIB_SvmStd_FLT ==
  pIn : Inport  OutDataTypeStr=Bus: SWLIBS_2Syst_FLT  BusOutputAsStruct=on
  GMCLIB_SvmStd_SF : S-Function  FunctionName=GMCLIB_SvmStd_SF_FLT  SFunctionDeploymentMode=off  EnableBusSupport=off
  copyright : Subsystem
      mask Display: text(10,90,'FILE:');text(10,75,'DESRIPTION:');text(10,60,'COPYRIGHT:');text(10,45,'VERSION:');text(10,30,'DATE:')
  copyright2 : Subsystem
      mask Display: text(10,90,'GMCLIB_SvmStd_BAM_FLT.mdl');text(10,75,'Standard Space Vector Modulation.');text(10,60,'NXP 2020');text(10,45,'1.0');text(10,30,'18-Mar-2020');
  u32Sector : Outport
  pOut : Outport  Port=2
  wires:
  GMCLIB_SvmStd_SF/2 -> pOut/1
  GMCLIB_SvmStd_SF/1 -> u32Sector/1
  pIn/1 -> GMCLIB_SvmStd_SF/1

== system ammclib_bam_S32K14x/GMCLIB/FLT/GMCLIB_SvmU0n_FLT ==
  pIn : Inport  OutDataTypeStr=Bus: SWLIBS_2Syst_FLT  BusOutputAsStruct=on
  GMCLIB_SvmU0n_SF : S-Function  FunctionName=GMCLIB_SvmU0n_SF_FLT  SFunctionDeploymentMode=off  EnableBusSupport=off
  copyright : Subsystem
      mask Display: text(10,90,'FILE:');text(10,75,'DESRIPTION:');text(10,60,'COPYRIGHT:');text(10,45,'VERSION:');text(10,30,'DATE:')
  copyright2 : Subsystem
      mask Display: text(10,90,'GMCLIB_SvmU0n_BAM_FLT.mdl');text(10,75,'Special Space Vector Modulation with O_000 Nulls.');text(10,60,'NXP 2020');text(10,45,'1.0');text(10,30,'18-Mar-2020');
  u32Sector : Outport
  pOut : Outport  Port=2
  wires:
  GMCLIB_SvmU0n_SF/2 -> pOut/1
  GMCLIB_SvmU0n_SF/1 -> u32Sector/1
  pIn/1 -> GMCLIB_SvmU0n_SF/1

== system ammclib_bam_S32K14x/GMCLIB/FLT/GMCLIB_SvmU7n_FLT ==
  pIn : Inport  OutDataTypeStr=Bus: SWLIBS_2Syst_FLT  BusOutputAsStruct=on
  GMCLIB_SvmU7n_SF : S-Function  FunctionName=GMCLIB_SvmU7n_SF_FLT  SFunctionDeploymentMode=off  EnableBusSupport=off
  copyright : Subsystem
      mask Display: text(10,90,'FILE:');text(10,75,'DESRIPTION:');text(10,60,'COPYRIGHT:');text(10,45,'VERSION:');text(10,30,'DATE:')
  copyright2 : Subsystem
      mask Display: text(10,90,'GMCLIB_SvmU7n_BAM_FLT.mdl');text(10,75,'Special Space Vector Modulation with O_111 Ones.');text(10,60,'NXP 2020');text(10,45,'1.0');text(10,30,'18-Mar-2020');
  u32Sector : Outport
  pOut : Outport  Port=2
  wires:
  GMCLIB_SvmU7n_SF/2 -> pOut/1
  GMCLIB_SvmU7n_SF/1 -> u32Sector/1
  pIn/1 -> GMCLIB_SvmU7n_SF/1

== system ammclib_bam_S32K14x/GMCLIB/FLT/GMCLIB_VRot_FLT ==
  fltInVec : Inport  OutDataTypeStr=Bus: SWLIBS_2Syst_FLT  BusOutputAsStruct=on
  fltAngle : Inport  Port=2  OutDataTypeStr=single
  GMCLIB_VRot_SF : S-Function  FunctionName=GMCLIB_VRot_SF_FLT  SFunctionDeploymentMode=off  EnableBusSupport=off
  copyright : Subsystem
      mask Display: text(10,90,'FILE:');text(10,75,'DESRIPTION:');text(10,60,'COPYRIGHT:');text(10,45,'VERSION:');text(10,30,'DATE:')
  copyright2 : Subsystem
      mask Display: text(10,90,'GMCLIB_VRot_BAM_FLT.mdl');text(10,75,'Vector rotation.');text(10,60,'NXP 2020');text(10,45,'1.0');text(10,30,'05-Jun-2020');
  fltOutVec : Outport
  wires:
  GMCLIB_VRot_SF/1 -> fltOutVec/1
  fltAngle/1 -> GMCLIB_VRot_SF/2
  fltInVec/1 -> GMCLIB_VRot_SF/1

== system ammclib_bam_S32K14x/GMCLIB/FLT/GMCLIB_VUnit_FLT ==
  fltInVec : Inport  OutDataTypeStr=Bus: SWLIBS_2Syst_FLT  BusOutputAsStruct=on
  GMCLIB_VUnit_SF : S-Function  FunctionName=GMCLIB_VUnit_SF_FLT  SFunctionDeploymentMode=off  EnableBusSupport=off
  copyright : Subsystem
      mask Display: text(10,90,'FILE:');text(10,75,'DESRIPTION:');text(10,60,'COPYRIGHT:');text(10,45,'VERSION:');text(10,30,'DATE:')
  copyright2 : Subsystem
      mask Display: text(10,90,'GMCLIB_VUnit_BAM_FLT.mdl');text(10,75,'Vector normalization.');text(10,60,'NXP 2020');text(10,45,'1.0');text(10,30,'08-Jun-2020');
  fltOutVec : Outport
  wires:
  GMCLIB_VUnit_SF/1 -> fltOutVec/1
  fltInVec/1 -> GMCLIB_VUnit_SF/1

== system ammclib_bam_S32K14x/GMCLIB/FLT/GMCLIB_Vpol2xy_FLT ==
  fltInVec : Inport  OutDataTypeStr=Bus: SWLIBS_2Syst_FLT  BusOutputAsStruct=on
  GMCLIB_Vpol2xy_SF : S-Function  FunctionName=GMCLIB_Vpol2xy_SF_FLT  SFunctionDeploymentMode=off  EnableBusSupport=off
  copyright : Subsystem
      mask Display: text(10,90,'FILE:');text(10,75,'DESRIPTION:');text(10,60,'COPYRIGHT:');text(10,45,'VERSION:');text(10,30,'DATE:')
  copyright2 : Subsystem
      mask Display: text(10,90,'GMCLIB_Vpol2xy_BAM_FLT.mdl');text(10,75,'Transformation of polar coordinate system to Cartesian.');text(10,60,'NXP 2020');text(10,45,'1.0');text(10,30,'10-Jun-2020');
  fltOutVec : Outport
  wires:
  GMCLIB_Vpol2xy_SF/1 -> fltOutVec/1
  fltInVec/1 -> GMCLIB_Vpol2xy_SF/1

== system ammclib_bam_S32K14x/GMCLIB/FLT/GMCLIB_Vxy2pol_FLT ==
  fltInVec : Inport  OutDataTypeStr=Bus: SWLIBS_2Syst_FLT  BusOutputAsStruct=on
  GMCLIB_Vxy2pol_SF : S-Function  FunctionName=GMCLIB_Vxy2pol_SF_FLT  SFunctionDeploymentMode=off  EnableBusSupport=off
  copyright : Subsystem
      mask Display: text(10,90,'FILE:');text(10,75,'DESRIPTION:');text(10,60,'COPYRIGHT:');text(10,45,'VERSION:');text(10,30,'DATE:')
  copyright2 : Subsystem
      mask Display: text(10,90,'GMCLIB_Vxy2pol_BAM_FLT.mdl');text(10,75,'Transformation of Cartesian coordinate system to polar.');text(10,60,'NXP 2020');text(10,45,'1.0');text(10,30,'11-Jun-2020');
  fltOutVec : Outport
  wires:
  GMCLIB_Vxy2pol_SF/1 -> fltOutVec/1
  fltInVec/1 -> GMCLIB_Vxy2pol_SF/1

== system ammclib_bam_S32K14x/MLIB/F16/MLIB_AbsSat_F16 ==
  f16In : Inport  OutDataTypeStr=int16
  MLIB_AbsSat_SF : S-Function  FunctionName=MLIB_AbsSat_SF_F16  SFunctionDeploymentMode=off  EnableBusSupport=off
  copyright : Subsystem
      mask Display: text(10,90,'FILE:');text(10,75,'DESRIPTION:');text(10,60,'COPYRIGHT:');text(10,45,'VERSION:');text(10,30,'DATE:')
  copyright2 : Subsystem
      mask Display: text(10,90,'MLIB_AbsSat_BAM_F16.mdl');text(10,75,'Saturated absolute value.');text(10,60,'NXP 2020');text(10,45,'1.0');text(10,30,'18-Mar-2020');
  f16Out : Outport
  wires:
  MLIB_AbsSat_SF/1 -> f16Out/1
  f16In/1 -> MLIB_AbsSat_SF/1

== system ammclib_bam_S32K14x/MLIB/F16/MLIB_Abs_F16 ==
  f16In : Inport  OutDataTypeStr=int16
  MLIB_Abs_SF : S-Function  FunctionName=MLIB_Abs_SF_F16  SFunctionDeploymentMode=off  EnableBusSupport=off
  copyright : Subsystem
      mask Display: text(10,90,'FILE:');text(10,75,'DESRIPTION:');text(10,60,'COPYRIGHT:');text(10,45,'VERSION:');text(10,30,'DATE:')
  copyright2 : Subsystem
      mask Display: text(10,90,'MLIB_Abs_BAM_F16.mdl');text(10,75,'Unsaturated absolute value.');text(10,60,'NXP 2020');text(10,45,'1.0');text(10,30,'18-Mar-2020');
  f16Out : Outport
  wires:
  MLIB_Abs_SF/1 -> f16Out/1
  f16In/1 -> MLIB_Abs_SF/1

== system ammclib_bam_S32K14x/MLIB/F16/MLIB_AddSat_F16 ==
  f16In1 : Inport  OutDataTypeStr=int16
  f16In2 : Inport  Port=2  OutDataTypeStr=int16
  MLIB_AddSat_SF : S-Function  FunctionName=MLIB_AddSat_SF_F16  SFunctionDeploymentMode=off  EnableBusSupport=off
  copyright : Subsystem
      mask Display: text(10,90,'FILE:');text(10,75,'DESRIPTION:');text(10,60,'COPYRIGHT:');text(10,45,'VERSION:');text(10,30,'DATE:')
  copyright2 : Subsystem
      mask Display: text(10,90,'MLIB_AddSat_BAM_F16.mdl');text(10,75,'Saturated addition.');text(10,60,'NXP 2020');text(10,45,'1.0');text(10,30,'18-Mar-2020');
  f16Out : Outport
  wires:
  MLIB_AddSat_SF/1 -> f16Out/1
  f16In2/1 -> MLIB_AddSat_SF/2
  f16In1/1 -> MLIB_AddSat_SF/1

== system ammclib_bam_S32K14x/MLIB/F16/MLIB_Add_F16 ==
  f16In1 : Inport  OutDataTypeStr=int16
  f16In2 : Inport  Port=2  OutDataTypeStr=int16
  MLIB_Add_SF : S-Function  FunctionName=MLIB_Add_SF_F16  SFunctionDeploymentMode=off  EnableBusSupport=off
  copyright : Subsystem
      mask Display: text(10,90,'FILE:');text(10,75,'DESRIPTION:');text(10,60,'COPYRIGHT:');text(10,45,'VERSION:');text(10,30,'DATE:')
  copyright2 : Subsystem
      mask Display: text(10,90,'MLIB_Add_BAM_F16.mdl');text(10,75,'Unsaturated addition.');text(10,60,'NXP 2020');text(10,45,'1.0');text(10,30,'18-Mar-2020');
  f16Out : Outport
  wires:
  MLIB_Add_SF/1 -> f16Out/1
  f16In2/1 -> MLIB_Add_SF/2
  f16In1/1 -> MLIB_Add_SF/1

== system ammclib_bam_S32K14x/MLIB/F16/MLIB_ConvertPU_F16F32 ==
  f32In : Inport  OutDataTypeStr=int32
  MLIB_ConvertPU_SF : S-Function  FunctionName=MLIB_ConvertPU_SF_F16F32  SFunctionDeploymentMode=off  EnableBusSupport=off
  copyright : Subsystem
      mask Display: text(10,90,'FILE:');text(10,75,'DESRIPTION:');text(10,60,'COPYRIGHT:');text(10,45,'VERSION:');text(10,30,'DATE:')
  copyright2 : Subsystem
      mask Display: text(10,90,'MLIB_ConvertPU_BAM_F16F32.mdl');text(10,75,'Converts the input value to a different representation.');text(10,60,'NXP 2020');text(10,45,'1.0');text(10,30,'18-Mar-2020');
  f16Out : Outport
  wires:
  MLIB_ConvertPU_SF/1 -> f16Out/1
  f32In/1 -> MLIB_ConvertPU_SF/1

== system ammclib_bam_S32K14x/MLIB/F16/MLIB_ConvertPU_F16FLT ==
  fltIn : Inport  OutDataTypeStr=single
  MLIB_ConvertPU_SF : S-Function  FunctionName=MLIB_ConvertPU_SF_F16FLT  SFunctionDeploymentMode=off  EnableBusSupport=off
  copyright : Subsystem
      mask Display: text(10,90,'FILE:');text(10,75,'DESRIPTION:');text(10,60,'COPYRIGHT:');text(10,45,'VERSION:');text(10,30,'DATE:')
  copyright2 : Subsystem
      mask Display: text(10,90,'MLIB_ConvertPU_BAM_F16FLT.mdl');text(10,75,'Converts the input value to a different representation.');text(10,60,'NXP 2020');text(10,45,'1.0');text(10,30,'18-Mar-2020');
  f16Out : Outport
  wires:
  MLIB_ConvertPU_SF/1 -> f16Out/1
  fltIn/1 -> MLIB_ConvertPU_SF/1

== system ammclib_bam_S32K14x/MLIB/F16/MLIB_Convert_F16F32 ==
  f32In1 : Inport  OutDataTypeStr=int32
  f32In2 : Inport  Port=2  OutDataTypeStr=int32
  MLIB_Convert_SF : S-Function  FunctionName=MLIB_Convert_SF_F16F32  SFunctionDeploymentMode=off  EnableBusSupport=off
  copyright : Subsystem
      mask Display: text(10,90,'FILE:');text(10,75,'DESRIPTION:');text(10,60,'COPYRIGHT:');text(10,45,'VERSION:');text(10,30,'DATE:')
  copyright2 : Subsystem
      mask Display: text(10,90,'MLIB_Convert_BAM_F16F32.mdl');text(10,75,'Converts the input value with scale to a different representation.');text(10,60,'NXP 2020');text(10,45,'1.0');text(10,30,'18-Mar-2020');
  f16Out : Outport
  wires:
  MLIB_Convert_SF/1 -> f16Out/1
  f32In2/1 -> MLIB_Convert_SF/2
  f32In1/1 -> MLIB_Convert_SF/1

== system ammclib_bam_S32K14x/MLIB/F16/MLIB_Convert_F16FLT ==
  fltIn1 : Inport  OutDataTypeStr=single
  fltIn2 : Inport  Port=2  OutDataTypeStr=single
  MLIB_Convert_SF : S-Function  FunctionName=MLIB_Convert_SF_F16FLT  SFunctionDeploymentMode=off  EnableBusSupport=off
  copyright : Subsystem
      mask Display: text(10,90,'FILE:');text(10,75,'DESRIPTION:');text(10,60,'COPYRIGHT:');text(10,45,'VERSION:');text(10,30,'DATE:')
  copyright2 : Subsystem
      mask Display: text(10,90,'MLIB_Convert_BAM_F16FLT.mdl');text(10,75,'Converts the input value with scale to a different representation.');text(10,60,'NXP 2020');text(10,45,'1.0');text(10,30,'18-Mar-2020');
  f16Out : Outport
  wires:
  MLIB_Convert_SF/1 -> f16Out/1
  fltIn2/1 -> MLIB_Convert_SF/2
  fltIn1/1 -> MLIB_Convert_SF/1

== system ammclib_bam_S32K14x/MLIB/F16/MLIB_DivSat_F16 ==
  f16In1 : Inport  OutDataTypeStr=int16
  f16In2 : Inport  Port=2  OutDataTypeStr=int16
  MLIB_DivSat_SF : S-Function  FunctionName=MLIB_DivSat_SF_F16  SFunctionDeploymentMode=off  EnableBusSupport=off
  copyright : Subsystem
      mask Display: text(10,90,'FILE:');text(10,75,'DESRIPTION:');text(10,60,'COPYRIGHT:');text(10,45,'VERSION:');text(10,30,'DATE:')
  copyright2 : Subsystem
      mask Display: text(10,90,'MLIB_DivSat_BAM_F16.mdl');text(10,75,'Saturated division.');text(10,60,'NXP 2020');text(10,45,'1.0');text(10,30,'18-Mar-2020');
  f16Out : Outport
  wires:
  MLIB_DivSat_SF/1 -> f16Out/1
  f16In2/1 -> MLIB_DivSat_SF/2
  f16In1/1 -> MLIB_DivSat_SF/1

== system ammclib_bam_S32K14x/MLIB/F16/MLIB_Div_F16 ==
  f16In1 : Inport  OutDataTypeStr=int16
  f16In2 : Inport  Port=2  OutDataTypeStr=int16
  MLIB_Div_SF : S-Function  FunctionName=MLIB_Div_SF_F16  SFunctionDeploymentMode=off  EnableBusSupport=off
  copyright : Subsystem
      mask Display: text(10,90,'FILE:');text(10,75,'DESRIPTION:');text(10,60,'COPYRIGHT:');text(10,45,'VERSION:');text(10,30,'DATE:')
  copyright2 : Subsystem
      mask Display: text(10,90,'MLIB_Div_BAM_F16.mdl');text(10,75,'Division of two input values.');text(10,60,'NXP 2020');text(10,45,'1.0');text(10,30,'18-Mar-2020');
  f16Out : Outport
  wires:
  MLIB_Div_SF/1 -> f16Out/1
  f16In2/1 -> MLIB_Div_SF/2
  f16In1/1 -> MLIB_Div_SF/1

== system ammclib_bam_S32K14x/MLIB/F16/MLIB_MacSat_F16 ==
  f16In1 : Inport  OutDataTypeStr=int16
  f16In2 : Inport  Port=2  OutDataTypeStr=int16
  f16In3 : Inport  Port=3  OutDataTypeStr=int16
  MLIB_MacSat_SF : S-Function  FunctionName=MLIB_MacSat_SF_F16  SFunctionDeploymentMode=off  EnableBusSupport=off
  copyright : Subsystem
      mask Display: text(10,90,'FILE:');text(10,75,'DESRIPTION:');text(10,60,'COPYRIGHT:');text(10,45,'VERSION:');text(10,30,'DATE:')
  copyright2 : Subsystem
      mask Display: text(10,90,'MLIB_MacSat_BAM_F16.mdl');text(10,75,'Saturated sum of two input values.');text(10,60,'NXP 2020');text(10,45,'1.0');text(10,30,'18-Mar-2020');
  f16Out : Outport
  wires:
  MLIB_MacSat_SF/1 -> f16Out/1
  f16In3/1 -> MLIB_MacSat_SF/3
  f16In2/1 -> MLIB_MacSat_SF/2
  f16In1/1 -> MLIB_MacSat_SF/1

== system ammclib_bam_S32K14x/MLIB/F16/MLIB_Mac_F16 ==
  f16In1 : Inport  OutDataTypeStr=int16
  f16In2 : Inport  Port=2  OutDataTypeStr=int16
  f16In3 : Inport  Port=3  OutDataTypeStr=int16
  MLIB_Mac_SF : S-Function  FunctionName=MLIB_Mac_SF_F16  SFunctionDeploymentMode=off  EnableBusSupport=off
  copyright : Subsystem
      mask Display: text(10,90,'FILE:');text(10,75,'DESRIPTION:');text(10,60,'COPYRIGHT:');text(10,45,'VERSION:');text(10,30,'DATE:')
  copyright2 : Subsystem
      mask Display: text(10,90,'MLIB_Mac_BAM_F16.mdl');text(10,75,'Multiply-accumulte.');text(10,60,'NXP 2020');text(10,45,'1.0');text(10,30,'18-Mar-2020');
  f16Out : Outport
  wires:
  MLIB_Mac_SF/1 -> f16Out/1
  f16In3/1 -> MLIB_Mac_SF/3
  f16In2/1 -> MLIB_Mac_SF/2
  f16In1/1 -> MLIB_Mac_SF/1

== system ammclib_bam_S32K14x/MLIB/F16/MLIB_Mnac_F16 ==
  f16In1 : Inport  OutDataTypeStr=int16
  f16In2 : Inport  Port=2  OutDataTypeStr=int16
  f16In3 : Inport  Port=3  OutDataTypeStr=int16
  MLIB_Mnac_SF : S-Function  FunctionName=MLIB_Mnac_SF_F16  SFunctionDeploymentMode=off  EnableBusSupport=off
  copyright : Subsystem
      mask Display: text(10,90,'FILE:');text(10,75,'DESRIPTION:');text(10,60,'COPYRIGHT:');text(10,45,'VERSION:');text(10,30,'DATE:')
  copyright2 : Subsystem
      mask Display: text(10,90,'MLIB_Mnac_BAM_F16.mdl');text(10,75,'Unsaturated multiply-negative-accumulate.');text(10,60,'NXP 2020');text(10,45,'1.0');text(10,30,'18-Mar-2020');
  f16Out : Outport
  wires:
  MLIB_Mnac_SF/1 -> f16Out/1
  f16In3/1 -> MLIB_Mnac_SF/3
  f16In2/1 -> MLIB_Mnac_SF/2
  f16In1/1 -> MLIB_Mnac_SF/1

== system ammclib_bam_S32K14x/MLIB/F16/MLIB_Msu_F16 ==
  f16In1 : Inport  OutDataTypeStr=int16
  f16In2 : Inport  Port=2  OutDataTypeStr=int16
  f16In3 : Inport  Port=3  OutDataTypeStr=int16
  MLIB_Msu_SF : S-Function  FunctionName=MLIB_Msu_SF_F16  SFunctionDeploymentMode=off  EnableBusSupport=off
  copyright : Subsystem
      mask Display: text(10,90,'FILE:');text(10,75,'DESRIPTION:');text(10,60,'COPYRIGHT:');text(10,45,'VERSION:');text(10,30,'DATE:')
  copyright2 : Subsystem
      mask Display: text(10,90,'MLIB_Msu_BAM_F16.mdl');text(10,75,'Unsaturated multiply-subtract-from.');text(10,60,'NXP 2020');text(10,45,'1.0');text(10,30,'18-Mar-2020');
  f16Out : Outport
  wires:
  MLIB_Msu_SF/1 -> f16Out/1
  f16In3/1 -> MLIB_Msu_SF/3
  f16In2/1 -> MLIB_Msu_SF/2
  f16In1/1 -> MLIB_Msu_SF/1

== system ammclib_bam_S32K14x/MLIB/F16/MLIB_MulSat_F16 ==
  f16In1 : Inport  OutDataTypeStr=int16
  f16In2 : Inport  Port=2  OutDataTypeStr=int16
  MLIB_MulSat_SF : S-Function  FunctionName=MLIB_MulSat_SF_F16  SFunctionDeploymentMode=off  EnableBusSupport=off
  copyright : Subsystem
      mask Display: text(10,90,'FILE:');text(10,75,'DESRIPTION:');text(10,60,'COPYRIGHT:');text(10,45,'VERSION:');text(10,30,'DATE:')
  copyright2 : Subsystem
      mask Display: text(10,90,'MLIB_MulSat_BAM_F16.mdl');text(10,75,'Saturated multiplication.');text(10,60,'NXP 2020');text(10,45,'1.0');text(10,30,'18-Mar-2020');
  f16Out : Outport
  wires:
  MLIB_MulSat_SF/1 -> f16Out/1
  f16In2/1 -> MLIB_MulSat_SF/2
  f16In1/1 -> MLIB_MulSat_SF/1

== system ammclib_bam_S32K14x/MLIB/F16/MLIB_Mul_F16 ==
  f16In1 : Inport  OutDataTypeStr=int16
  f16In2 : Inport  Port=2  OutDataTypeStr=int16
  MLIB_Mul_SF : S-Function  FunctionName=MLIB_Mul_SF_F16  SFunctionDeploymentMode=off  EnableBusSupport=off
  copyright : Subsystem
      mask Display: text(10,90,'FILE:');text(10,75,'DESRIPTION:');text(10,60,'COPYRIGHT:');text(10,45,'VERSION:');text(10,30,'DATE:')
  copyright2 : Subsystem
      mask Display: text(10,90,'MLIB_Mul_BAM_F16.mdl');text(10,75,'Unsaturated multiplication.');text(10,60,'NXP 2020');text(10,45,'1.0');text(10,30,'18-Mar-2020');
  f16Out : Outport
  wires:
  MLIB_Mul_SF/1 -> f16Out/1
  f16In2/1 -> MLIB_Mul_SF/2
  f16In1/1 -> MLIB_Mul_SF/1
